simulink model "ILnormal2k18"  (R2018a)
settings: Solver=FixedStepAuto  StartTime=0.0  StopTime=10  FixedStep=0.1  RelTol=1e-3
libraries: simulink x4
settings Model: Creator=training  LastModifiedBy=training
settings DataIOCC: ReturnWorkspaceOutputs=on
settings SFSimCC: SimUseLocalCustomCode=on
settings RTWCC: RTWUseLocalCustomCode=on

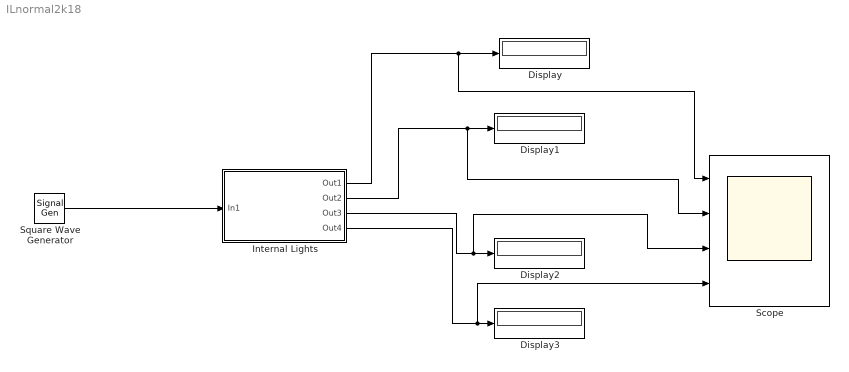
== system ILnormal2k18 ==
  Display{,1..3} (4 alike) : Display
  Internal Lights : Subsystem
  Scope : Scope  NumInputPorts=4
  Square Wave Generator : SignalGenerator  WaveForm=square  Units=rad/sec
  wires:
  Square Wave Generator/1 -> Internal Lights/1(In1)
  Internal Lights/1(Out1) -> Scope/1, Display/1
  Internal Lights/2(Out2) -> Scope/2, Display1/1
  Internal Lights/3(Out3) -> Scope/3, Display2/1
  Internal Lights/4(Out4) -> Scope/4, Display3/1

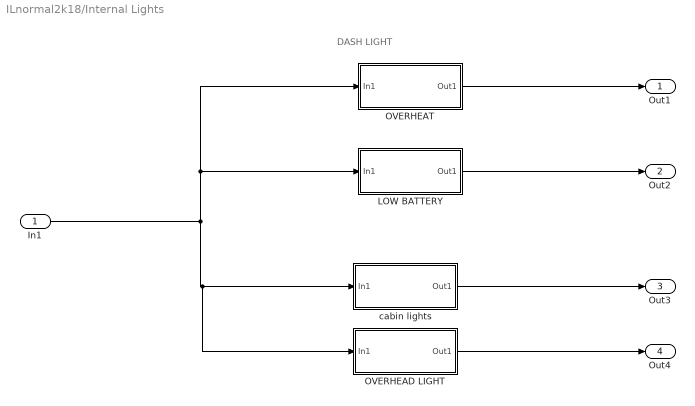
== system ILnormal2k18/Internal Lights ==
  note: DASH LIGHT
  In1 : Inport
  LOW BATTERY : Subsystem
  OVERHEAD LIGHT : Subsystem
  OVERHEAT : Subsystem
  cabin lights : Subsystem
  Out1 : Outport
  Out2 : Outport  Port=2
  Out3 : Outport  Port=3
  Out4 : Outport  Port=4
  wires:
  In1/1 -> OVERHEAD LIGHT/1(In1), cabin lights/1(In1), LOW BATTERY/1(In1), OVERHEAT/1(In1)
  OVERHEAT/1(Out1) -> Out1/1
  LOW BATTERY/1(Out1) -> Out2/1
  OVERHEAD LIGHT/1(Out1) -> Out4/1
  cabin lights/1(Out1) -> Out3/1

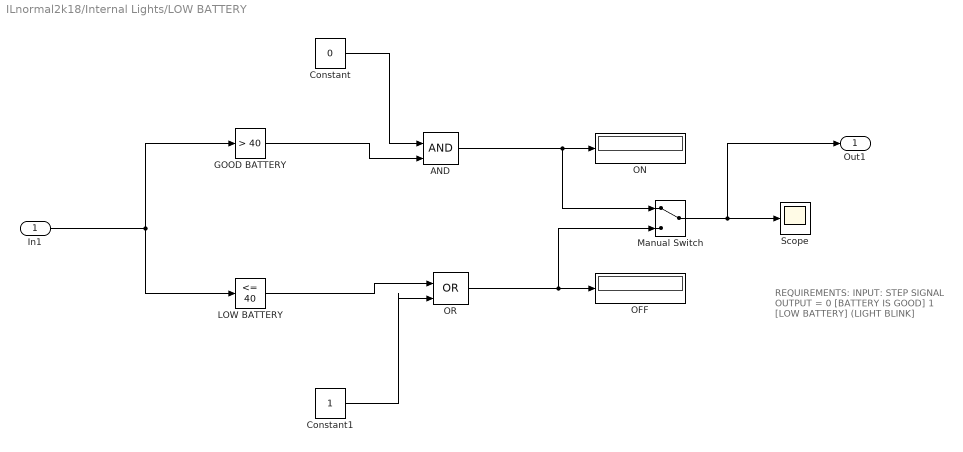
== system ILnormal2k18/Internal Lights/LOW BATTERY ==
  note: REQUIREMENTS:
      | INPUT: STEP SIGNAL
      | OUTPUT = 0 [BATTERY IS GOOD]
      | 1 [LOW BATTERY] (LIGHT BLINK]
  In1 : Inport
  AND : Logic  IconShape=distinctive  AllPortsSameDT=off  OutDataTypeStr=boolean
  Constant : Constant  Value=0
  Constant1 : Constant
  GOOD BATTERY : simulink/Logic and Bit Operations/Compare To Constant  relop=>  const=40  OutDataTypeStr=boolean
  LOW BATTERY : simulink/Logic and Bit Operations/Compare To Constant  relop=<=  const=40  OutDataTypeStr=boolean
  Manual Switch : ManualSwitch
  OFF : Display
  ON : Display
  OR : Logic  Operator=OR  IconShape=distinctive  AllPortsSameDT=off  OutDataTypeStr=boolean
  Scope : Scope
  Out1 : Outport
  wires:
  OR/1 -> Manual Switch/2, OFF/1
  AND/1 -> Manual Switch/1, ON/1
  Manual Switch/1 -> Out1/1, Scope/1
  Constant1/1 -> OR/2
  GOOD BATTERY/1 -> AND/2
  Constant/1 -> AND/1
  LOW BATTERY/1 -> OR/1
  In1/1 -> LOW BATTERY/1, GOOD BATTERY/1

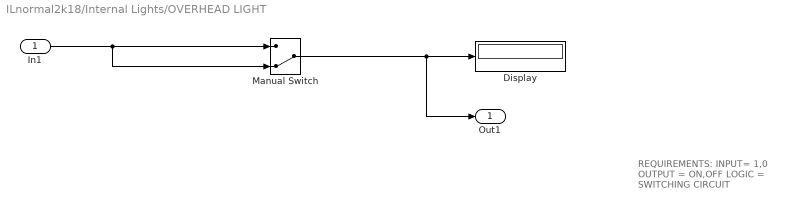
== system ILnormal2k18/Internal Lights/OVERHEAD LIGHT ==
  note: REQUIREMENTS:
      | INPUT= 1,0
      | OUTPUT = ON,OFF
      | LOGIC = SWITCHING CIRCUIT
  In1 : Inport
  Display : Display
  Manual Switch : ManualSwitch  CurrentSetting=0
  Out1 : Outport
  wires:
  In1/1 -> Manual Switch/2, Manual Switch/1
  Manual Switch/1 -> Out1/1, Display/1

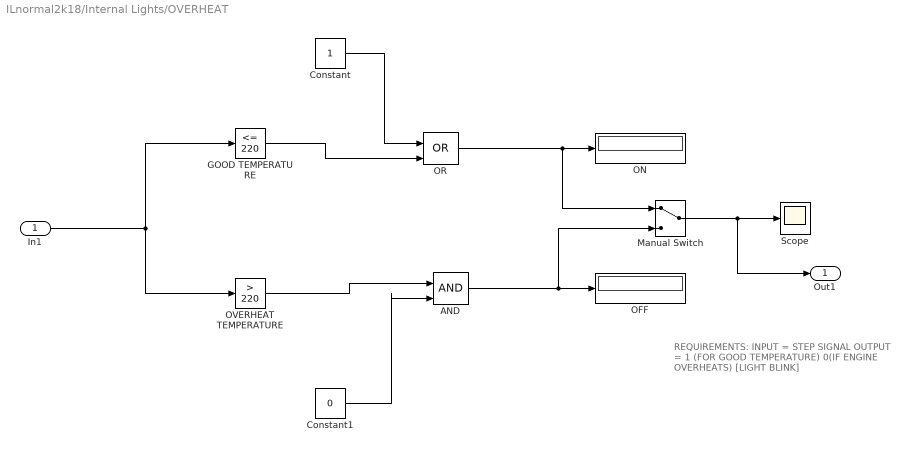
== system ILnormal2k18/Internal Lights/OVERHEAT ==
  note: REQUIREMENTS:
      | INPUT = STEP SIGNAL
      | OUTPUT = 1 (FOR GOOD TEMPERATURE)
      | 0(IF ENGINE OVERHEATS) [LIGHT BLINK]
  In1 : Inport
  AND : Logic  IconShape=distinctive  AllPortsSameDT=off  OutDataTypeStr=boolean
  Constant : Constant
  Constant1 : Constant  Value=0
  GOOD TEMPERATURE : simulink/Logic and Bit Operations/Compare To Constant  relop=<=  const=220  OutDataTypeStr=boolean
  Manual Switch : ManualSwitch
  OFF : Display
  ON : Display
  OR : Logic  Operator=OR  IconShape=distinctive  AllPortsSameDT=off  OutDataTypeStr=boolean
  OVERHEAT TEMPERATURE : simulink/Logic and Bit Operations/Compare To Constant  relop=>  const=220  OutDataTypeStr=boolean
  Scope : Scope
  Out1 : Outport
  wires:
  In1/1 -> OVERHEAT TEMPERATURE/1, GOOD TEMPERATURE/1
  Constant/1 -> OR/1
  GOOD TEMPERATURE/1 -> OR/2
  OVERHEAT TEMPERATURE/1 -> AND/1
  Constant1/1 -> AND/2
  OR/1 -> Manual Switch/1, ON/1
  AND/1 -> Manual Switch/2, OFF/1
  Manual Switch/1 -> Out1/1, Scope/1

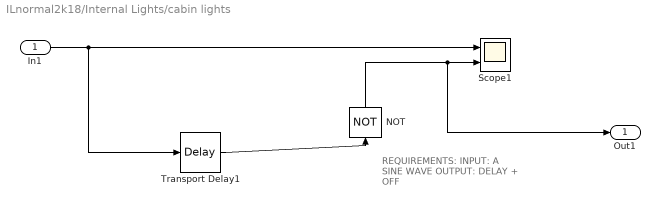
== system ILnormal2k18/Internal Lights/cabin lights ==
  note: REQUIREMENTS:
      | INPUT: A SINE WAVE
      | OUTPUT: DELAY + OFF
  In1 : Inport
  NOT : Logic  Operator=NOT  AllPortsSameDT=off  OutDataTypeStr=boolean
  Scope1 : Scope  NumInputPorts=2
  Transport Delay1 : TransportDelay  DelayTime=3
  Out1 : Outport
  wires:
  Transport Delay1/1 -> NOT/1
  NOT/1 -> Out1/1, Scope1/2
  In1/1 -> Scope1/1, Transport Delay1/1
